simulink model "festo_control_Unity_finger_angle_nosensor"  (R2021a)
settings: Solver=VariableStepAuto  StartTime=0.0  StopTime=inf  RelTol=1e-3
model workspace (MATLAB code in the model file):
  | %config file for Matlab server for Matlab-unity communication
  | portPi = 12345;
  | %%%THIS PART IS INPUT THAT IS OK TO CHANGE TO YOUR NEEDS%%%
  | IPAddress = '127.0.0.1';                            %address for Matlab-Unity communication. 127.0.0.1 means local
  | portNr = 26950;                                     %make sure that this port matches the one chosen in Unity
  | nrMessages = 3;                                     %nr of values that you are reading in per packet. Depends on your Unity settings
  | sampleFrequency = 500;                              %frequency on Simulink checking TCP connection
  | 
  | %%%THIS PART YOU ONLY HAVE TO TOUCH WHEN THE UNITY MESSAGE TYPE OR HEADER CHANGES%%
  | headerWidth = 12;                                   %nr of bytes in message header (before actual message)
  | signalWidth = 8;                                    %length of each value in message, depends on data type (which is double for now, which is 8 bytes)
  | messageWidth = nrMessages .* signalWidth;           %length of message without header
  | totalMessageWidth = headerWidth + messageWidth;     %length of total packet
  | sampleTime = 1/sampleFrequency;
libraries: slrealtimeutilitieslib x4, slrealtimeiplib x2, instrumentlib x1
settings Model: EnablePacing=on  Creator=slacker  LastModifiedBy=20210123
settings SolverCC: AlgebraicLoopSolver=TrustRegion
settings DebuggingCC: SFMachineParentedDataDiag=warning

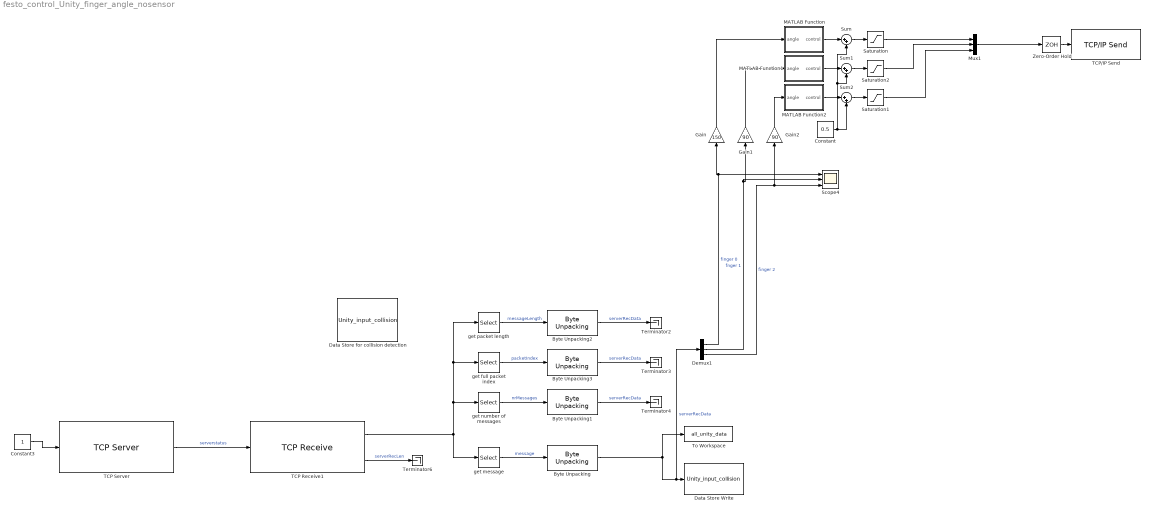
== system festo_control_Unity_finger_angle_nosensor ==
  Byte Unpacking{,1..3} (4 alike) : slrealtimeutilitieslib/Byte Unpacking
      settings: SourceProductBaseCode=XP
  Constant : Constant  Value=0.5
  Constant3 : Constant  OutDataTypeStr=double
  Data Store Write : DataStoreWrite  DataStoreName=Unity_input_collision  DataStoreElements=Unity_input_collision  IndexOptions=Index vector (port)  Indices=1  OutputSizes=1
  Data Store for collision detection : DataStoreMemory  DataStoreName=Unity_input_collision  ReadBeforeWriteMsg=warning  WriteAfterWriteMsg=warning  WriteAfterReadMsg=warning  InitialValue=zeros(1,nrMessages)  ShowAdditionalParam=off
  Demux1 : Demux  Outputs=3
  Gain : Gain  Gain=150
  Gain1 : Gain  Gain=90
  Gain2 : Gain  Gain=90
  MATLAB Function : MATLAB Function  TreatAsAtomicUnit=on
  MATLAB Function1 : MATLAB Function  TreatAsAtomicUnit=on
  MATLAB Function2 : MATLAB Function  TreatAsAtomicUnit=on
  Mux1 : Mux  Inputs=3
  Saturation : Saturate  UpperLimit=0.7  LowerLimit=0
  Saturation1 : Saturate  UpperLimit=0.7  LowerLimit=0
  Saturation2 : Saturate  UpperLimit=0.7  LowerLimit=0
  Scope4 : Scope  NumInputPorts=3
  Sum : Sum  Inputs=|++
  Sum1 : Sum  Inputs=|++
  Sum2 : Sum  Inputs=|++
  TCP Receive1 : slrealtimeiplib/TCP Receive  socketAddPortVal=Server: IPAddress:portNr  rcvWidth=totalMessageWidth  sampleTime=sampleTime
      settings: SourceProductBaseCode=XP
  TCP Server : slrealtimeiplib/TCP Server  Priority=-1  useHostTargetConn=off  serverAddress=IPAddress  serverPort=portNr
      settings: SourceProductBaseCode=XP
  TCP/IP Send : instrumentlib/TCP//IP Send  Host=131.155.162.21  Port=12346  EnableBlockingMode=on  Timeout=0.5  ByteOrder=LittleEndian  TransferDelay=on
  Terminator{2..4,6} (4 alike) : Terminator
  To Workspace : ToWorkspace  VariableName=all_unity_data  SaveFormat=Timeseries  SampleTime=-1
  Zero-Order Hold : ZeroOrderHold  SampleTime=0.004
  get full packet index : Selector  InputPortWidth=totalMessageWidth  IndexOptions=Index vector (dialog)  Indices=[5:8]  OutputSizes=1
  get message : Selector  InputPortWidth=totalMessageWidth  IndexOptions=Index vector (dialog)  Indices=[headerWidth+1:totalMessageWidth]  OutputSizes=1
  get number of messages : Selector  InputPortWidth=totalMessageWidth  IndexOptions=Index vector (dialog)  Indices=[9:headerWidth]  OutputSizes=1
  get packet length : Selector  InputPortWidth=totalMessageWidth  IndexOptions=Index vector (dialog)  Indices=[1:4]  OutputSizes=1
  wires:
  Saturation/1 -> Mux1/1
  Mux1/1 -> Zero-Order Hold/1
  Zero-Order Hold/1 -> TCP/IP Send/1
  Saturation1/1 -> Mux1/3
  Saturation2/1 -> Mux1/2
  get number of messages/1 -> Byte Unpacking1/1  "nrMessages"
  get full packet index/1 -> Byte Unpacking3/1  "packetIndex"
  TCP Receive1/2 -> Terminator6/1  "serverRecLen"
  Byte Unpacking2/1 -> Terminator2/1  "serverRecData"
  get packet length/1 -> Byte Unpacking2/1  "messageLength"
  TCP Receive1/1 -> get message/1, get number of messages/1, get full packet index/1, get packet length/1
  Byte Unpacking/1 -> Demux1/1, Data Store Write/1, To Workspace/1  "serverRecData"
  Byte Unpacking3/1 -> Terminator3/1  "serverRecData"
  Byte Unpacking1/1 -> Terminator4/1  "serverRecData"
  TCP Server/1 -> TCP Receive1/1  "serverstatus"
  get message/1 -> Byte Unpacking/1  "message"
  Constant3/1 -> TCP Server/1
  Demux1/3 -> Gain2/1, Scope4/3  "finger 2"
  Demux1/2 -> Gain1/1, Scope4/2  "fnger 1"
  Demux1/1 -> Gain/1, Scope4/1  "finger 0"
  MATLAB Function/1(control) -> Sum/1
  Sum/1 -> Saturation/1
  MATLAB Function1/1(control) -> Sum1/1
  Sum1/1 -> Saturation2/1
  MATLAB Function2/1(control) -> Sum2/1
  Sum2/1 -> Saturation1/1
  Constant/1 -> Sum2/2, Sum/2, Sum1/2
  Gain/1 -> MATLAB Function/1(angle)
  Gain1/1 -> MATLAB Function1/1(angle)
  Gain2/1 -> MATLAB Function2/1(angle)

== matlab function festo_control_Unity_finger_angle_nosensor/MATLAB Function ==
  data: angle input; control output
function control = angleToControl(angle)
    p1 =        5684;
    p2 =      -164.2;
    p3 =       1.004;
    delta = p2^2-4*p1*(p3-angle);
    x1 = (-p2+sqrt(delta))/(2*p1);
    x2 = (-p2-sqrt(delta))/(2*p1);
    if x1 <= 0.5 && x1 >=0
        control = x1;
    elseif x2 <= 0.5 && x2 >=0
        control = x2;
    else
        control = 0;
    end
end

== matlab function festo_control_Unity_finger_angle_nosensor/MATLAB Function2 ==
  data: angle input; control output
function control = angleToControl(angle)
    p1 =        5684;
    p2 =      -164.2;
    p3 =       1.004;
    delta = p2^2-4*p1*(p3-angle);
    x1 = (-p2+sqrt(delta))/(2*p1);
    x2 = (-p2-sqrt(delta))/(2*p1);
    if x1 <= 0.5 && x1 >=0
        control = x1;
    elseif x2 <= 0.5 && x2 >=0
        control = x2;
    else
        control = 0;
    end
end

== matlab function festo_control_Unity_finger_angle_nosensor/MATLAB Function1 ==
  data: angle input; control output
function control = angleToControl(angle)
    p1 =        5684;
    p2 =      -164.2;
    p3 =       1.004;
    delta = p2^2-4*p1*(p3-angle);
    x1 = (-p2+sqrt(delta))/(2*p1);
    x2 = (-p2-sqrt(delta))/(2*p1);
    if x1 <= 0.5 && x1 >=0
        control = x1;
    elseif x2 <= 0.5 && x2 >=0
        control = x2;
    else
        control = 0;
    end
end
